simulink model "DJI_Quadcopter_Simulation_2018a"  (R2018a)
settings: Solver=ode45  StartTime=0  StopTime=40  FixedStep=0.02  MaxStep=0.06  RelTol=1e-3  EnableMultiTasking=on
InitFcn:
  | load('batteryModelNew.mat');
  | load('soc_ocv_new.mat');
  | 
  | Q      = battery.QParam; % total capacity in mAh
  | n       = battery.etaParam; % coulombic efficiency
  | M      = battery.MParam; % dynamic hysteresis volts factor
  | Mo     = battery.M0Param; % instant hysteresis volts factor
  | Ro     = battery.R0Param; % internal resistance
  | R       = [battery.RCParam(1)]; % diffusion / warburg impedence, pairs with C
  | C       = [battery.RCParam(2)]; % diffusion / warburg impedence, pairs with R
  | g       = battery.GParam;  % gamma, tunes decay in hysteresis
  | dt      = .01; % delta t
  | eod   = battery.EODParam; % final voltage
  | 
  | if length(R) ~= length(C)
  |     error("R and C must be the same length");
  | end
  | 
  | Arc = zeros(length(R));
  | for i = 1:length(R)
  |     Arc(i,i) = exp(-dt/(R(i)*C(i)));
  | end
  | Brc = zeros(length(R), 1);
  | for i = 1:length(R)
  |     Brc(i,1) = 1 - exp(-dt/(R(i)*C(i)));
  | end
  | k = 1; % timestep
  | Io = .1; % current at time k
  | H(k) = exp(-abs((n(k)*Io(k)*g*dt)/Q));
  | 
  | 
  | %Io = current(1:floor(length(current)/2.5));
  | %Io = current;
  | Io = 0.0;
  | 
  | z = 1.0; % soc
  | Ir = zeros(length(R), 1);
  | h = 0.0;
  | v = ones(length(Io));
  | 
  | 
  | soc = zeros(1, length(Io));
  | v = soc;
model workspace (MAT data in the model file):
  Sig = Simulink.Signal
  Sig.DataType = 'auto'
  Sig.Dimensions = -1
  Sig.DimensionsMode = 'auto'
  Sig.Complexity = 'auto'
  Sig.SampleTime = -1
  Sig.SamplingMode = 'auto'
undefined symbols (not defined in the file): IC, Motor, quadModel, soc_ocv
libraries: simulink x5
(part 1 of 2)
Description:
  | This is a configurable quadcopter simulation.
  | This Simulink model demonstates attitude control.
  | 
  | Additional quadcopter modeling and simulation materials available at:
  | github.com/dch33/Quad-Sim
  | 
  | Copyright (C) 2014 D. Hartman, K. Landis, S. Moreno, J. Kim, M. Mehrer
  | 
  | License:
  |     This program is free software: you can redistribute it and/or modify
  |     it under the terms of the GNU LESSER GENERAL PUBLIC LICENSE as published by
  |     the Free Software Foundation, either version 3 of the License, or
  |     (at your option) any later version.
  | 
  |     This program is distributed in the hope that it will be useful,
  |     but WITHOUT ANY WARRANTY; without even the implied warranty of
  |     MERCHANTABILITY or FITNESS FOR A PARTICULAR PURPOSE.  See the
  |     GNU General Public License for more details.
  | 
  |     You should have received a copy of the GNU LESSER GENERAL PUBLIC LICENSE
  |     along with this program.  If not, see <http://www.gnu.org/licenses/>.
settings Model: ModifiedComment=tdarrah -- Tue Jun 04 05:29:55 2019 -- Version 1.39  Creator=David Hartman  LastModifiedBy=tdarrah
settings Model: ModifiedHistory=|
  | tdarrah -- Tue Jun 04 05:29:55 2019 -- Version 1.39
  | 
  | tdarrah -- Tue Jun 04 05:29:55 2019 -- Version 1.39
  | 
  | tdarrah -- Mon Jun 03 18:31:35 2019 -- Version 1.38
  | closed the battery loop
  | 
  | tdarrah -- Mon Jun 03 18:20:30 2019 -- Version 1.37
  | added battery
  | 
  | 
  | tdarrah -- Mon Jun 03 17:58:08 2019 -- Version 1.36
  | incorporated our motors in model
  | 
  | 
  | Sahai Couso -- Fri May 10 11:35:12 2019 -- Version 1.35
  | 
  | Sahai Couso -- Fri May 10 10:41:34 2019 -- Version 1.34
  | 
  | Sahai Couso -- Fri May 10 10:40:52 2019 -- Version 1.33
  | 
  | Sahai Couso -- Fri May 10 10:30:50 2019 -- Version 1.32
  | 
  | Sahai Couso -- Fri May 10 10:24:25 2019 -- Version 1.31
  | 
  | Sahai Couso -- Wed May 08 22:16:35 2019 -- Version 1.30
  | 
  | Sahai Couso -- Wed May 08 22:15:23 2019 -- Version 1.29
  | 
  | Sahai Couso -- Wed May 08 22:14:58 2019 -- Version 1.28
  | 
  | Sahai Couso -- Wed May 08 22:04:36 2019 -- Version 1.27
  | 
  | Sahai Couso -- Wed May 08 22:04:16 2019 -- Version 1.26
  | 
  | Sahai Couso -- Wed May 08 21:57:14 2019 -- Version 1.25
  | 
  | Sahai Couso -- Wed May 08 21:54:04 2019 -- Version 1.24
  | 
  | Sahai Couso -- Wed May 08 21:53:17 2019 -- Version 1.23
  | 
  | Sahai Couso -- Wed May 08 21:48:07 2019 -- Version 1.22
  | 
  | Sahai Couso -- Wed May 08 21:35:53 2019 -- Version 1.21
  | 
  | Sahai Couso -- Wed May 08 21:28:21 2019 -- Version 1.19
  | 
  | Sahai Couso -- Wed May 08 21:28:21 2019 -- Version 1.19
  | 
  | Sahai Couso -- Wed May 08 21:25:30 2019 -- Version 1.18
  | 
  | Sahai Couso -- Wed May 08 21:23:06 2019 -- Version 1.17
  | 
  | Sahai Couso -- Wed May 08 13:57:34 2019 -- Version 1.16
  | 
  | Sahai Couso -- Wed May 08 00:58:43 2019 -- Version 1.15
  | 
  | Sahai Couso -- Wed May 08 00:58:03 2019 -- Version 1.14
  | 
  | Sahai Couso -- Tue May 07 23:55:58 2019 -- Version 1.13
  | 
  | Sahai Couso -- Tue May 07 23:08:00 2019 -- Version 1.12
  | 
  | Sahai Couso -- Tue May 07 23:06:52 2019 -- Version 1.11
  | 
  | Sahai Couso -- Tue May 07 22:57:09 2019 -- Version 1.10
  | 
  | Sahai Couso -- Tue May 07 22:48:57 2019 -- Version 1.9
  | 
  | Sahai Couso -- Tue May 07 21:40:08 2019 -- Version 1.8
  | 
  | Yves -- Tue Apr 04 13:12:37 2017 -- Version 1.7
  | 
  | Yves -- Tue Apr 04 13:10:33 2017 -- Version 1.6
  | 
  | davidhartman -- Fri Jun 06 23:19:51 2014 -- Version 1.5
  | 
  | 
  | davidhartman -- Fri Jun 06 22:53:10 2014 -- Version 1.3
settings SolverCC: AutoInsertRateTranBlk=on
settings DataIOCC: SaveFormat=Array  SignalLogging=off
settings OptimizationCC: DefaultParameterBehavior=Inlined  LifeSpan=inf
settings DebuggingCC: UnderspecifiedInitializationDetection=Classic  MergeDetectMultiDrivingBlocksExec=none  SolverPrmCheckMsg=warning  UniqueDataStoreMsg=warning  StateNameClashWarn=warning  StrictBusMsg=WarnOnBusTreatedAsVector  SFUnexpectedBacktrackingDiag=warning  SFNoUnconditionalDefaultTransitionDiag=warning  SFExecutionAtInitializationDiag=none
settings HardwareCC: ProdBitPerPointer=32  ProdBitPerSizeT=32  ProdBitPerPtrDiffT=32  ProdLargestAtomicFloat=None  ProdIntDivRoundTo=Undefined  ProdEndianess=Unspecified  ProdWordSize=32  ProdHWDeviceType=32-bit Generic
settings ModelReferenceCC: PropagateSignalLabelsOutOfModel=off
settings CodeAppCC: StateflowObjectComments=on
settings GRTTargetCC: TargetLangStandard=C89/C90 (ANSI)  GeneratePreprocessorConditionals=Disable all
settings ConfigComp: CovMetricSettings=dw  CovHtmlReporting=on  CovSaveCumulativeToWorkspaceVar=on  CovSaveSingleToWorkspaceVar=on  CovExternalEMLEnable=off

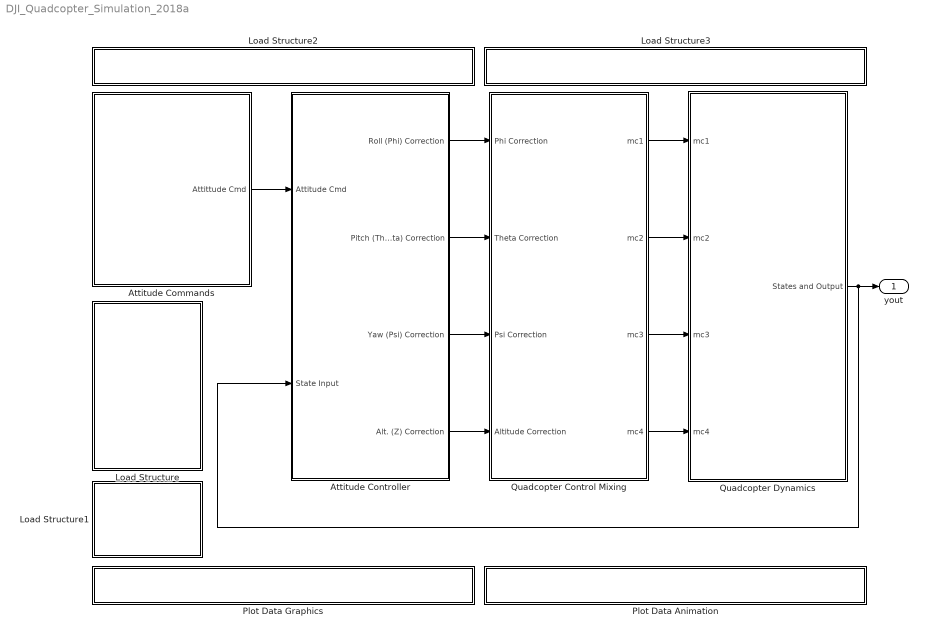
== system DJI_Quadcopter_Simulation_2018a ==
  Attitude Commands : Subsystem
  Attitude Controller : Subsystem
  Load Structure : Subsystem
      settings: OpenFcn=|
      | uiopen('load')
      | if (exist('IC')==1 && exist('quadModel')==1)
      | set_param(bdroot, 'SimulationCommand', 'update')
      | end
      mask Display: fprintf('LOAD:\nQuadcopter\nModel Or\nInitial\nConditions');
  Load Structure1 : Subsystem
      settings: OpenFcn=|
      | if (exist('IC')==1 && exist('quadModel')==1 && exist('yout') && exist('tout'))
      | saveSimResults()
      | else
      | msgbox('No Data To Save!')
      | end
      mask Display: fprintf('SAVE:\nSimulation\nResults');
  Load Structure2 : Subsystem
      settings: OpenFcn=|
      | if exist('GUI_Modeling') == 2,
      | run('GUI_Modeling')
      | 
      | else
      | 
      | msgbox('The desired GUI must be first added to MATLABs path.')
      | 
      | end
      mask Display: fprintf('OPEN GUI: Build New \n Model');
  Load Structure3 : Subsystem
      settings: OpenFcn=|
      | if exist('GUI_IC') == 2,
      | run('GUI_IC')
      | 
      | else
      | 
      | msgbox('The desired GUI must be first added to MATLABs path.')
      | 
      | end
      mask Display: fprintf('OPEN GUI: Create Initial \n Conditions');
  Plot Data Animation : Subsystem
      settings: OpenFcn=|
      | if exist('QuadAnim4') == 2,
      |     if exist('yout')
      | 	run('QuadAnim4');
      |     else
      |     msgbox('Simulation must be run before data can be plotted.');
      |     end
      | else                                                                          msgbox('The desired GUI must be first added to MATLABs path.')
      | end
      mask Display: fprintf('OPEN GUI: Flight Animation')
  Plot Data Graphics : Subsystem
      settings: OpenFcn=|
      | if exist('yout')
      | yout = evalin('base', 'yout');
      | tout = evalin('base', 'tout');
      | quadPlots(yout, tout)
      | else
      | msgbox('Simulation must be run before data can be plotted.')
      | end
      mask Display: fprintf('OPEN PLOT: State Data')
  Quadcopter Control Mixing : Subsystem
      mask Display:
      | modelLoaded = evalin('base','exist(''quadModel'',''var'')');
      | if (modelLoaded==1)
      |     if (evalin('base','quadModel.plusConfig'))
      |     fprintf([' \n' ' \n'  'Configuration "+"']);
      |     else if (~evalin('base','quadModel.plusConfig'))
      |         fprintf([' \n' ' \n' 'Configuration "X"']);
      |         end
      |     end
      | else
      |     fprintf([' \n' ' \n'  'Model Not Loaded']);
      | end
  Quadcopter Dynamics : Subsystem
  yout : Outport
  wires:
  Quadcopter Dynamics/1(States and Output) -> yout/1, Attitude Controller/2(State Input)
  Quadcopter Control Mixing/1(mc1) -> Quadcopter Dynamics/1(mc1)
  Quadcopter Control Mixing/2(mc2) -> Quadcopter Dynamics/2(mc2)
  Quadcopter Control Mixing/3(mc3) -> Quadcopter Dynamics/3(mc3)
  Quadcopter Control Mixing/4(mc4) -> Quadcopter Dynamics/4(mc4)
  Attitude Controller/1(Roll (Phi) Correction) -> Quadcopter Control Mixing/1(Phi Correction)
  Attitude Controller/2(Pitch (Theta) Correction) -> Quadcopter Control Mixing/2(Theta Correction)
  Attitude Controller/3(Yaw (Psi) Correction) -> Quadcopter Control Mixing/3(Psi Correction)
  Attitude Controller/4(Alt. (Z) Correction) -> Quadcopter Control Mixing/4(Altitude Correction)
  Attitude Commands/1(Attittude Cmd) -> Attitude Controller/1(Attitude Cmd)

== system DJI_Quadcopter_Simulation_2018a/Attitude Commands ==
  Bus Creator : BusCreator  Inputs=4
  Step : Step  Time=4  After=-10*pi/180  SampleTime=0
  Step1 : Step  After=10*pi/180  SampleTime=0
  Step2 : Step  Time=7  After=45*pi/180  SampleTime=0
  Step3 : Step  Time=0  Before=10*0.3048  After=10*0.3048  SampleTime=0
  Attittude Cmd : Outport
  tag scope: A=global
  wires:
  Bus Creator/1 -> Attittude Cmd/1, [A]  "Attitude_Cmd"
  Step3/1 -> Bus Creator/4  "Alt_cmd"
  Step2/1 -> Bus Creator/3  "Psi_cmd"
  Step1/1 -> Bus Creator/2  "The_cmd"
  Step/1 -> Bus Creator/1  "Phi_cmd"

== system DJI_Quadcopter_Simulation_2018a/Attitude Controller ==
  Attitude Cmd : Inport
  State Input : Inport  Port=2
  Altitude (Z) Control : Subsystem  mask{Kpz=2, Kiz=1.1, Kdz=3.3, LimitOutput=on, USat=1, LSat=-1, GOffset=(sqrt((quadModel.mass*quadModel.g)/(4*quadModel.ct))-quadModel.b)/quadModel.cr}
      mask prompts: Kpz "Kp"; Kiz "Ki"; Kdz "Kd"; LimitOutput "Integral Saturation?"; USat "Upper saturation limit:"; LSat "Lower saturation limit:"; GOffset "Gravity Feedforward"
      mask help:
      | Adjust PID controller gains through this mask interface, or "look under mask" for more detailed adjustments.
      |
      | Note: Gravity Offset will not appear on block face as a value until simulation is run if it is the result of a formula involving the quadcopter model parameters.
      mask TypeOptions Kpz: Kpz/Gain
      mask TypeOptions Kiz: Kiz/Gain
      mask TypeOptions Kdz: Kdz/Gain
      mask TypeOptions LimitOutput:
      | Integrator
      | Limited/LimitOutput
      mask TypeOptions USat:
      | Integrator
      | Limited/UpperSaturationLimit
      mask TypeOptions LSat:
      | Integrator
      | Limited/LowerSaturationLimit
      mask TypeOptions GOffset: Gravity Offset (Level Flight)/Value
      mask Display:
      | fprintf(['Gravity Offset = ' num2str(GOffset) '\n' ...
      |     'Kp = ' num2str(Kpz) '\n' ...
      |     'Ki = ' num2str(Kiz) '\n' ...
      |     'Kd = ' num2str(Kdz) '\n' ...
      |     'Integral Saturation: ' LimitOutput]);
      | if strcmp(LimitOutput,'on')
      |     fprintf([' \n' ' \n' ' \n' ' \n' ' \n' '\n' ...
      |         'Limits: ' num2str(USat) ' to ' num2str(LSat)]);
      | end
  Bus Selector : BusSelector  OutputSignals=Phi,P,The,Q,Psi,R,Z
  Pitch (Theta) Control : Subsystem  mask{Kpt=2, Kit=1.1, Kdt=1.2, LimitOutput=on, USat=1, LSat=-1}
      mask prompts: Kpt "Kp"; Kit "Ki"; Kdt "Kd"; LimitOutput "Integral Saturation?"; USat "Upper saturation limit:"; LSat "Lower saturation limit:"
      mask help: Adjust PID controller gains through this mask interface, or "look under mask" for more detailed adjustments.
      mask TypeOptions Kpt: Kpt/Gain
      mask TypeOptions Kit: Kit/Gain
      mask TypeOptions Kdt: Kdt/Gain
      mask TypeOptions LimitOutput:
      | Integrator
      | Limited/LimitOutput
      mask TypeOptions USat:
      | Integrator
      | Limited/UpperSaturationLimit
      mask TypeOptions LSat:
      | Integrator
      | Limited/LowerSaturationLimit
      mask Display:
      | fprintf(['Kp = ' num2str(Kpt) '\n' ...
      |     'Ki = ' num2str(Kit) '\n' ...
      |     'Kd = ' num2str(Kdt) '\n' ...
      |     'Integral Saturation: ' LimitOutput]);
      | if strcmp(LimitOutput,'on')
      |     fprintf([' \n' ' \n' ' \n' ' \n' '\n' ...
      |         'Limits: ' num2str(USat) ' to ' num2str(LSat)]);
      | end
  "Roll (Phi) Control " : Subsystem  mask{Kpp=2.0, Kip=1.1, Kdp=1.2, LimitOutput=on, USat=1, LSat=-1}
      mask prompts: Kpp "Kp"; Kip "Ki"; Kdp "Kd"; LimitOutput "Integral Saturation:"; USat "Upper saturation limit:"; LSat "Lower saturation limit:"
      mask help:
      | Adjust PID controller gains through this mask interface, or "look under mask"
      | for more detailed adjustments.
      mask TypeOptions Kpp: Kpp/Gain
      mask TypeOptions Kip: Kip/Gain
      mask TypeOptions Kdp: Kdp/Gain
      mask TypeOptions LimitOutput:
      | Integrator
      | Limited/LimitOutput
      mask TypeOptions USat:
      | Integrator
      | Limited/UpperSaturationLimit
      mask TypeOptions LSat:
      | Integrator
      | Limited/LowerSaturationLimit
      mask Display:
      | fprintf(['Kp = ' num2str(Kpp) '\n' ...
      |     'Ki = ' num2str(Kip) '\n' ...
      |     'Kd = ' num2str(Kdp) '\n'...
      |     'Integral Saturation: ' LimitOutput]);
      | if strcmp(LimitOutput,'on')
      |     fprintf([' \n' ' \n' ' \n' ' \n' '\n' ...
      |         'Limits: ' num2str(USat) ' to ' num2str(LSat)]);
      | end
  Yaw (Psi) Control : Subsystem  mask{Kps=4, Kis=0.5, Kds=3.5, LimitOutput=on, USat=1, LSat=-1}
      mask prompts: Kps "Kp"; Kis "Ki"; Kds "Kd"; LimitOutput "Integral Saturation?"; USat "Upper saturation limit:"; LSat "Lower saturation limit:"
      mask help: Adjust PID controller gains through this mask interface, or "look under mask" for more detailed adjustments.
      mask TypeOptions Kps: Kps/Gain
      mask TypeOptions Kis: Kit/Gain
      mask TypeOptions Kds: Kds/Gain
      mask TypeOptions LimitOutput:
      | Integrator
      | Limited/LimitOutput
      mask TypeOptions USat:
      | Integrator
      | Limited/UpperSaturationLimit
      mask TypeOptions LSat:
      | Integrator
      | Limited/LowerSaturationLimit
      mask Display:
      | fprintf(['Kp = ' num2str(Kps) '\n' ...
      |     'Ki = ' num2str(Kis) '\n' ...
      |     'Kd = ' num2str(Kds) '\n' ...
      |     'Integral Saturation: ' LimitOutput]);
      | if strcmp(LimitOutput,'on')
      |     fprintf([' \n' ' \n' ' \n' ' \n' '\n' ...
      |         'Limits: ' num2str(USat) ' to ' num2str(LSat)]);
      | end
  Roll (Phi) Correction : Outport
  Pitch (Theta) Correction : Outport  Port=2
  Yaw (Psi) Correction : Outport  Port=3
  Alt. (Z) Correction : Outport  Port=4
  wires:
  Bus Selector/6 -> Yaw (Psi) Control/3(R State)  "<R>"
  Bus Selector/4 -> Pitch (Theta) Control/3(Q State)  "<Q>"
  Bus Selector/2 -> "Roll (Phi) Control "/3(P)  "<P>"
  Bus Selector/3 -> Pitch (Theta) Control/2(Theta State)  "<The>"
  Attitude Cmd/1 -> "Roll (Phi) Control "/1("Attitude Command "), Pitch (Theta) Control/1(Attitude Command), Yaw (Psi) Control/1(Attitude Command), Altitude (Z) Control/1(Desired Z)
  Bus Selector/7 -> Altitude (Z) Control/2(Z State)  "<Z>"
  Altitude (Z) Control/1(Alt. (Z) Correction) -> Alt. (Z) Correction/1
  Bus Selector/5 -> Yaw (Psi) Control/2(Psi State)  "<Psi>"
  Yaw (Psi) Control/1(Psi Correction) -> Yaw (Psi) Correction/1
  Pitch (Theta) Control/1(Theta Correction) -> Pitch (Theta) Correction/1
  State Input/1 -> Bus Selector/1
  Bus Selector/1 -> "Roll (Phi) Control "/2(Phi State)  "<Phi>"
  "Roll (Phi) Control "/1(Phi Correction) -> Roll (Phi) Correction/1

== system DJI_Quadcopter_Simulation_2018a/Load Structure ==

== system DJI_Quadcopter_Simulation_2018a/Load Structure1 ==

== system DJI_Quadcopter_Simulation_2018a/Load Structure2 ==

== system DJI_Quadcopter_Simulation_2018a/Load Structure3 ==

== system DJI_Quadcopter_Simulation_2018a/Plot Data Animation ==

== system DJI_Quadcopter_Simulation_2018a/Plot Data Graphics ==

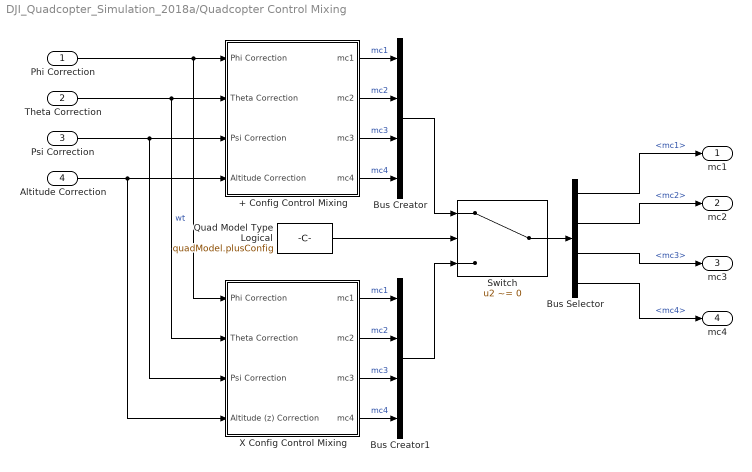
== system DJI_Quadcopter_Simulation_2018a/Quadcopter Control Mixing ==
  Phi Correction : Inport
  Theta Correction : Inport  Port=2
  Psi Correction : Inport  Port=3
  Altitude Correction : Inport  Port=4
  + Config Control Mixing : Subsystem
  Bus Creator : BusCreator  Inputs=4
  Bus Creator1 : BusCreator  Inputs=4
  Bus Selector : BusSelector  OutputSignals=mc1,mc2,mc3,mc4
  Quad Model Type Logical : Constant  Value=quadModel.plusConfig
  Switch : Switch  Criteria=u2 ~= 0
  X Config Control Mixing : Subsystem
  mc1 : Outport
  mc2 : Outport  Port=2
  mc3 : Outport  Port=3
  mc4 : Outport  Port=4
  wires:
  Switch/1 -> Bus Selector/1
  Quad Model Type Logical/1 -> Switch/2
  Bus Selector/4 -> mc4/1  "<mc4>"
  Bus Selector/3 -> mc3/1  "<mc3>"
  Bus Selector/2 -> mc2/1  "<mc2>"
  Bus Selector/1 -> mc1/1  "<mc1>"
  Bus Creator1/1 -> Switch/3
  X Config Control Mixing/4(mc4) -> Bus Creator1/4  "mc4"
  X Config Control Mixing/3(mc3) -> Bus Creator1/3  "mc3"
  X Config Control Mixing/2(mc2) -> Bus Creator1/2  "mc2"
  X Config Control Mixing/1(mc1) -> Bus Creator1/1  "mc1"
  Bus Creator/1 -> Switch/1
  + Config Control Mixing/4(mc4) -> Bus Creator/4  "mc4"
  + Config Control Mixing/3(mc3) -> Bus Creator/3  "mc3"
  + Config Control Mixing/2(mc2) -> Bus Creator/2  "mc2"
  + Config Control Mixing/1(mc1) -> Bus Creator/1  "mc1"
  Altitude Correction/1 -> + Config Control Mixing/4(Altitude Correction), X Config Control Mixing/4(Altitude (z) Correction)
  Psi Correction/1 -> + Config Control Mixing/3(Psi Correction), X Config Control Mixing/3(Psi Correction)
  Theta Correction/1 -> + Config Control Mixing/2(Theta Correction), X Config Control Mixing/2(Theta Correction)  "wt"
  Phi Correction/1 -> + Config Control Mixing/1(Phi Correction), X Config Control Mixing/1(Phi Correction)

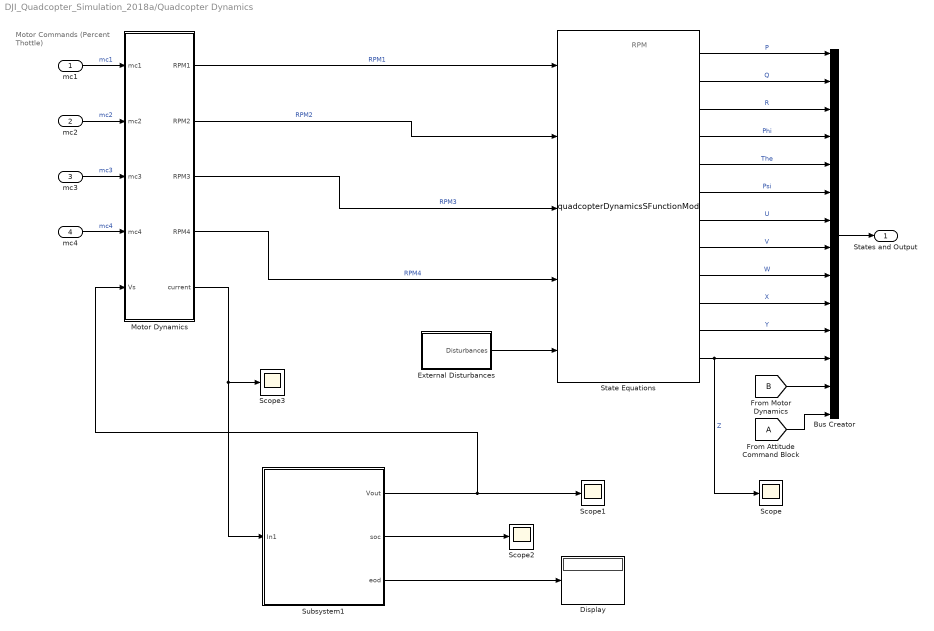
== system DJI_Quadcopter_Simulation_2018a/Quadcopter Dynamics ==
  note: Motor Commands
      | (Percent Thottle)
  note: RPM
  mc1 : Inport
  mc2 : Inport  Port=2
  mc3 : Inport  Port=3
  mc4 : Inport  Port=4
  Bus Creator : BusCreator  Inputs='P','Q','R','Phi','The','Psi','U','V','W','X','Y','Z','mc and RPM','Attitude_Cmd'
  Display : Display
  External Disturbances : Subsystem
  Motor Dynamics : Subsystem
  Scope{,1..3} (4 alike) : Scope
  State Equations : M-S-Function  FunctionName=quadcopterDynamicsSFunctionMod  Parameters=quadModel, IC
      mask Display:
      | port_label('input', 1, 'RPM1')
      | port_label('input', 2, 'RPM2')
      | port_label('input', 3, 'RPM3')
      | port_label('input', 4, 'RPM4')
      | port_label('input', 5, 'Disturbances')
      | port_label('output', 1, 'P')
      | port_label('output', 2, 'Q')
      | port_label('output', 3, 'R')
      | port_label('output', 4, 'Phi')
      | port_label('output', 5, 'The')
      | port_label('output', 6, 'Psi')
      | port_label('output', 7, 'U')
      | port_label('output', 8, 'V')
      | port_label('output', 9, 'W')
      | port_label('output', 10, 'X')
      | port_label('output', 11, 'Y')
      | port_label('output', 12, 'Z')
  Subsystem1 : Subsystem
  States and Output : Outport
  wires:
  [B] -> Bus Creator/13
  [A] -> Bus Creator/14
  External Disturbances/1("Disturbances ") -> State Equations/5
  mc2/1 -> Motor Dynamics/2(mc2)  "mc2"
  mc3/1 -> Motor Dynamics/3(mc3)  "mc3"
  mc4/1 -> Motor Dynamics/4(mc4)  "mc4"
  mc1/1 -> Motor Dynamics/1(mc1)  "mc1"
  Motor Dynamics/4(RPM4) -> State Equations/4  "RPM4"
  Motor Dynamics/3(RPM3) -> State Equations/3  "RPM3"
  Motor Dynamics/2(RPM2) -> State Equations/2  "RPM2"
  Motor Dynamics/1(RPM1) -> State Equations/1  "RPM1"
  Bus Creator/1 -> States and Output/1
  State Equations/12 -> Scope/1, Bus Creator/12  "Z"
  State Equations/11 -> Bus Creator/11  "Y"
  State Equations/10 -> Bus Creator/10  "X"
  State Equations/9 -> Bus Creator/9  "W"
  State Equations/8 -> Bus Creator/8  "V"
  State Equations/7 -> Bus Creator/7  "U"
  State Equations/6 -> Bus Creator/6  "Psi"
  State Equations/5 -> Bus Creator/5  "The"
  State Equations/4 -> Bus Creator/4  "Phi"
  State Equations/3 -> Bus Creator/3  "R"
  State Equations/2 -> Bus Creator/2  "Q"
  State Equations/1 -> Bus Creator/1  "P"
  Subsystem1/1(Vout) -> Motor Dynamics/5(Vs), Scope1/1
  Subsystem1/2(soc) -> Scope2/1
  Subsystem1/3(eod) -> Display/1
  Motor Dynamics/5(current) -> Scope3/1, Subsystem1/1(In1)

== system DJI_Quadcopter_Simulation_2018a/Attitude Controller/Altitude (Z) Control ==
  note: ez
  note: Improve to use rotation matrix and euler angles...
      | maybe with saturation?
  Desired Z : Inport
  Z State : Inport  Port=2
  Bus Selector : BusSelector  OutputSignals=Alt_cmd
  Derivative : Derivative
  Gravity Offset (Level Flight) : Constant  Value=GOffset
  Integrator Limited : Integrator  LimitOutput=on  UpperSaturationLimit=USat  LowerSaturationLimit=LSat
  Kdz : Gain  Gain=Kdz
  Kiz : Gain  Gain=Kiz
  Kpz : Gain  Gain=Kpz
  Scope : Scope
  Scope1 : Scope
  Scope2 : Scope
  Sum : Sum  Inputs=|+-
  Sum2 : Sum  Inputs=+++-
  Alt. (Z) Correction : Outport
  wires:
  Derivative/1 -> Kdz/1
  Bus Selector/1 -> Sum/1  "<Alt_cmd>"
  Integrator Limited/1 -> Kiz/1
  Kdz/1 -> Sum2/4  "D Corr"
  Kiz/1 -> Sum2/3  "I Corr"
  Sum/1 -> Scope/1, Kpz/1, Integrator Limited/1  "Error"
  Kpz/1 -> Sum2/2  "P Corr"
  Sum2/1 -> Scope1/1, Alt. (Z) Correction/1
  Z State/1 -> Sum/2, Derivative/1
  Desired Z/1 -> Bus Selector/1
  Gravity Offset (Level Flight)/1 -> Scope2/1, Sum2/1

== system DJI_Quadcopter_Simulation_2018a/Attitude Controller/Pitch (Theta) Control ==
  Attitude Command : Inport
  Theta State : Inport  Port=2
  Q State : Inport  Port=3
  Bus Selector : BusSelector  OutputSignals=The_cmd
  Integrator Limited : Integrator  LimitOutput=on  UpperSaturationLimit=USat  LowerSaturationLimit=LSat
  Kdt : Gain  Gain=Kdt
  Kit : Gain  Gain=Kit
  Kpt : Gain  Gain=Kpt
  Sum : Sum  Inputs=|+-
  Sum1 : Sum  Inputs=++-
  Theta Correction : Outport
  wires:
  Q State/1 -> Kdt/1
  Bus Selector/1 -> Sum/1  "<The_cmd>"
  Integrator Limited/1 -> Kit/1
  Kit/1 -> Sum1/2  "I Corr"
  Kdt/1 -> Sum1/3  "D Corr"
  Kpt/1 -> Sum1/1  "P Corr"
  Sum1/1 -> Theta Correction/1
  Theta State/1 -> Sum/2
  Attitude Command/1 -> Bus Selector/1
  Sum/1 -> Kpt/1, Integrator Limited/1  "Error"

== system DJI_Quadcopter_Simulation_2018a/Attitude Controller/Roll (Phi) Control  ==
  "Attitude Command " : Inport
  Phi State : Inport  Port=2
  P : Inport  Port=3
  Bus Selector : BusSelector  OutputSignals=Phi_cmd
  Integrator Limited : Integrator  LimitOutput=on  UpperSaturationLimit=USat  LowerSaturationLimit=LSat
  Kdp : Gain  Gain=Kdp
  Kip : Gain  Gain=Kip
  Kpp : Gain  Gain=Kpp
  Sum : Sum  Inputs=|+-
  Sum1 : Sum  Inputs=++-
  Phi Correction : Outport
  wires:
  P/1 -> Kdp/1
  Bus Selector/1 -> Sum/1  "<Phi_cmd>"
  "Attitude Command "/1 -> Bus Selector/1
  Integrator Limited/1 -> Kip/1
  Kip/1 -> Sum1/2  "I Corr"
  Kdp/1 -> Sum1/3  "D Corr"
  Kpp/1 -> Sum1/1  "P Corr"
  Sum1/1 -> Phi Correction/1
  Phi State/1 -> Sum/2
  Sum/1 -> Kpp/1, Integrator Limited/1  "Error"

== system DJI_Quadcopter_Simulation_2018a/Attitude Controller/Yaw (Psi) Control ==
  Attitude Command : Inport
  Psi State : Inport  Port=2
  R State : Inport  Port=3
  Bus Selector : BusSelector  OutputSignals=Psi_cmd
  Integrator Limited : Integrator  LimitOutput=on  UpperSaturationLimit=USat  LowerSaturationLimit=LSat
  Kds : Gain  Gain=Kds
  Kit : Gain  Gain=Kis
  Kps : Gain  Gain=Kps
  Sum : Sum  Inputs=|+-
  Sum1 : Sum  Inputs=++-
  Psi Correction : Outport
  wires:
  R State/1 -> Kds/1
  Bus Selector/1 -> Sum/1  "<Psi_cmd>"
  Integrator Limited/1 -> Kit/1
  Kit/1 -> Sum1/2  "I Corr"
  Kds/1 -> Sum1/3  "D Corr"
  Kps/1 -> Sum1/1  "P Corr"
  Psi State/1 -> Sum/2
  Sum1/1 -> Psi Correction/1
  Attitude Command/1 -> Bus Selector/1
  Sum/1 -> Kps/1, Integrator Limited/1  "Error"

== system DJI_Quadcopter_Simulation_2018a/Quadcopter Control Mixing/+ Config Control Mixing ==
  note: mc1 = Alt_cor -Psi_cor - The_cor
  note: mc3 = Alt_cor - Psi_cor + The_cor
  note: mc4 = Alt_cor + Psi_cor - Phi_cor
  note: + (plus) Quad Configuration Control Mixing
  note: mc2 = Alt_cor + Psi_cor + Phi_cor
  Phi Correction : Inport
  Theta Correction : Inport  Port=2
  Psi Correction : Inport  Port=3
  Altitude Correction : Inport  Port=4
  Sum1 : Sum  Inputs=|+-
  Sum11 : Sum  Inputs=-+|
  Sum2 : Sum  Inputs=|+-
  Sum3 : Sum  Inputs=++|
  Sum4 : Sum  Inputs=++|
  Sum8 : Sum  Inputs=|++
  mc1 : Outport
  mc2 : Outport  Port=2
  mc3 : Outport  Port=3
  mc4 : Outport  Port=4
  wires:
  Sum11/1 -> mc4/1
  Sum8/1 -> mc2/1
  Sum3/1 -> mc3/1
  Sum1/1 -> mc1/1
  Phi Correction/1 -> Sum11/1, Sum8/2
  Sum4/1 -> Sum8/1, Sum11/2
  Psi Correction/1 -> Sum2/2, Sum4/1
  Sum2/1 -> Sum1/1, Sum3/2
  Altitude Correction/1 -> Sum4/2, Sum2/1
  Theta Correction/1 -> Sum3/1, Sum1/2

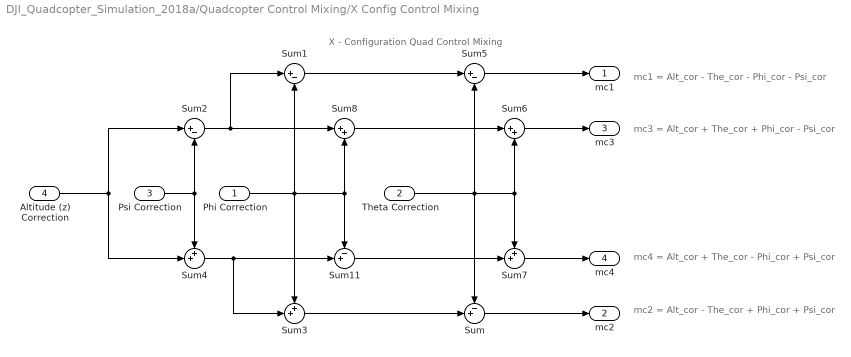
== system DJI_Quadcopter_Simulation_2018a/Quadcopter Control Mixing/X Config Control Mixing ==
  note: mc4 = Alt_cor + The_cor - Phi_cor + Psi_cor
  note: mc2 = Alt_cor - The_cor + Phi_cor + Psi_cor
  note: mc3 = Alt_cor + The_cor + Phi_cor - Psi_cor
  note: X - Configuration Quad Control Mixing
  note: mc1 = Alt_cor - The_cor - Phi_cor - Psi_cor
  Phi Correction : Inport
  Theta Correction : Inport  Port=2
  Psi Correction : Inport  Port=3
  Altitude (z) Correction : Inport  Port=4
  Sum : Sum  Inputs=-+|
  Sum1 : Sum  Inputs=|+-
  Sum11 : Sum  Inputs=-+|
  Sum2 : Sum  Inputs=|+-
  Sum3 : Sum  Inputs=++|
  Sum4 : Sum  Inputs=++|
  Sum5 : Sum  Inputs=|+-
  Sum6 : Sum  Inputs=|++
  Sum7 : Sum  Inputs=++|
  Sum8 : Sum  Inputs=|++
  mc1 : Outport
  mc2 : Outport  Port=2
  mc3 : Outport  Port=3
  mc4 : Outport  Port=4
  wires:
  Sum/1 -> mc2/1
  Altitude (z) Correction/1 -> Sum4/2, Sum2/1
  Sum7/1 -> mc4/1
  Sum6/1 -> mc3/1
  Sum5/1 -> mc1/1
  Sum11/1 -> Sum7/2
  Sum8/1 -> Sum6/1
  Sum1/1 -> Sum5/1
  Theta Correction/1 -> Sum/1, Sum5/2, Sum6/2, Sum7/1
  Sum3/1 -> Sum/2
  Sum4/1 -> Sum11/2, Sum3/2
  Phi Correction/1 -> Sum11/1, Sum8/2, Sum1/2, Sum3/1
  Psi Correction/1 -> Sum2/2, Sum4/1
  Sum2/1 -> Sum1/1, Sum8/1

== system DJI_Quadcopter_Simulation_2018a/Quadcopter Dynamics/External Disturbances ==
  note: Note: Torques are in units of N*m, Forces in N
      | Torques are applied to the BODY coordinate system.
      | Forces are applied from the WORLD coordinate system!
      | This can be changed by adjusting the equations within the S-function.
  Bus Creator : BusCreator  Inputs=6
  Bus to Vector : BusToVector
  Constant{2..6} (5 alike) : Constant  Value=0
  Step : Step  After=0  SampleTime=0
  "Disturbances " : Outport
  wires:
  Constant5/1 -> Bus Creator/6  "Force_z-axis"
  Constant4/1 -> Bus Creator/5  "Force_y-axis"
  Constant3/1 -> Bus Creator/4  "Force_x-axis"
  Constant2/1 -> Bus Creator/3  "Tau_bz-axis"
  Step/1 -> Bus Creator/2  "Tau_by-axis"
  Constant6/1 -> Bus Creator/1  "Tau_bx-axis"
  Bus Creator/1 -> Bus to Vector/1
  Bus to Vector/1 -> "Disturbances "/1

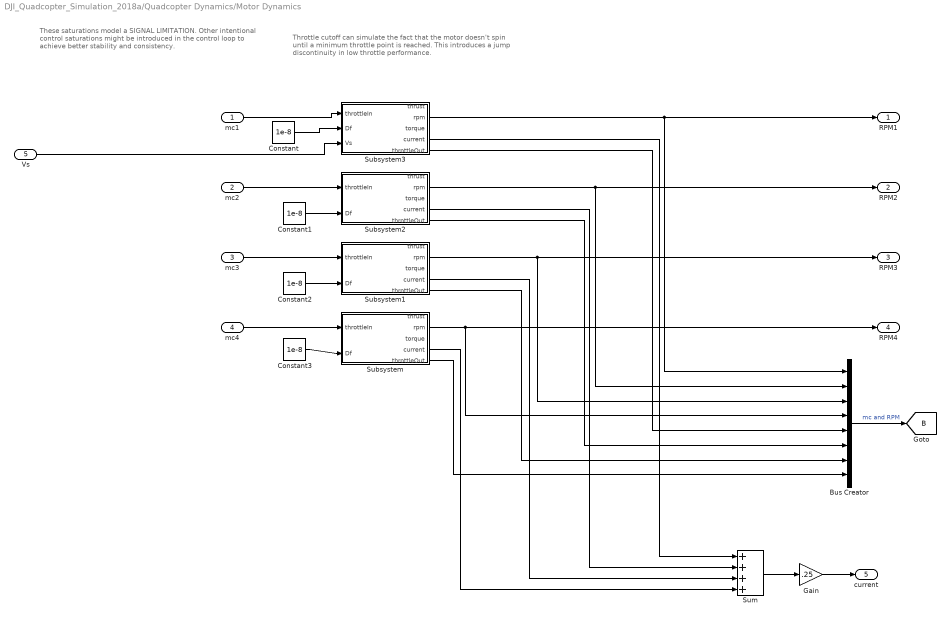
== system DJI_Quadcopter_Simulation_2018a/Quadcopter Dynamics/Motor Dynamics ==
  note: These saturations model a SIGNAL LIMITATION.
      | Other intentional control saturations might be introduced in the
      | control loop to achieve better stability and consistency.
  note: Throttle cutoff can simulate the fact that the motor doesn't
      | spin until a minimum throttle point is reached. This introduces
      | a jump discontinuity in low throttle performance.
  mc1 : Inport
  mc2 : Inport  Port=2
  mc3 : Inport  Port=3
  mc4 : Inport  Port=4
  Vs : Inport  Port=5
  Bus Creator : BusCreator  Inputs=8
  Constant{,1..3} (4 alike) : Constant  Value=1e-8
  Gain : Gain  Gain=.25
  Subsystem : Subsystem
  Subsystem1 : Subsystem
  Subsystem2 : Subsystem
  Subsystem3 : Subsystem
  Sum : Sum  Inputs=++++
  RPM1 : Outport
  RPM2 : Outport  Port=2
  RPM3 : Outport  Port=3
  RPM4 : Outport  Port=4
  current : Outport  Port=5
  tag scope: B=global
  wires:
  Bus Creator/1 -> [B]  "mc and RPM"
  Subsystem3/2(rpm) -> RPM1/1, Bus Creator/1
  mc1/1 -> Subsystem3/1(throttleIn)
  Constant/1 -> Subsystem3/2(Df)
  Subsystem3/5(throttleOut) -> Bus Creator/5
  Subsystem2/2(rpm) -> RPM2/1, Bus Creator/2
  mc2/1 -> Subsystem2/1(throttleIn)
  Constant1/1 -> Subsystem2/2(Df)
  Subsystem2/5(throttleOut) -> Bus Creator/6
  Subsystem1/2(rpm) -> Bus Creator/3, RPM3/1
  mc3/1 -> Subsystem1/1(throttleIn)
  Constant2/1 -> Subsystem1/2(Df)
  Subsystem1/5(throttleOut) -> Bus Creator/7
  Subsystem/2(rpm) -> RPM4/1, Bus Creator/4
  mc4/1 -> Subsystem/1(throttleIn)
  Constant3/1 -> Subsystem/2(Df)
  Subsystem/5(throttleOut) -> Bus Creator/8
  Subsystem/4(current) -> Sum/4
  Subsystem1/4(current) -> Sum/3
  Subsystem2/4(current) -> Sum/2
  Subsystem3/4(current) -> Sum/1
  Sum/1 -> Gain/1
  Vs/1 -> Subsystem3/3(Vs)
  Gain/1 -> current/1

== system DJI_Quadcopter_Simulation_2018a/Quadcopter Dynamics/Subsystem1 ==
  In1 : Inport
  Constant1 : Constant  Value=0
  Display1 : Display
  Equal : RelationalOperator  Operator===  OutDataTypeStr=boolean  RndMeth=Simplest
  Scope3 : Scope
  Stop Simulation : Stop
  Subsystem : Subsystem
  Vout : Outport
  soc : Outport  Port=2
  eod : Outport  Port=3
  wires:
  Subsystem/1(Vout) -> Vout/1
  Subsystem/2(soc) -> soc/1
  In1/1 -> Equal/1, Scope3/1, Subsystem/1(current)
  Subsystem/3(eod) -> eod/1
  Constant1/1 -> Equal/2
  Equal/1 -> Display1/1, Stop Simulation/1

== system DJI_Quadcopter_Simulation_2018a/Quadcopter Dynamics/Motor Dynamics/Subsystem ==
  throttleIn : Inport
  Df : Inport  Port=2
  Signal_Saturation_4 : Saturate  UpperLimit=100  LowerLimit=0
  Throttle To RPM Gain and Cutoff_8 : Subsystem
  motorRotor4 : Subsystem
  thrust : Outport
  rpm : Outport  Port=2
  torque : Outport  Port=3
  current : Outport  Port=4
  throttleOut : Outport  Port=5
  wires:
  Throttle To RPM Gain and Cutoff_8/1(Out5) -> motorRotor4/1(V)
  motorRotor4/4(current) -> current/1
  motorRotor4/2(rpm) -> rpm/1
  throttleIn/1 -> Signal_Saturation_4/1
  motorRotor4/3(torque) -> torque/1
  motorRotor4/1(thrust) -> thrust/1
  Signal_Saturation_4/1 -> Throttle To RPM Gain and Cutoff_8/1(In5), throttleOut/1
  Df/1 -> motorRotor4/2(Df)

== system DJI_Quadcopter_Simulation_2018a/Quadcopter Dynamics/Motor Dynamics/Subsystem1 ==
  throttleIn : Inport
  Df : Inport  Port=2
  Signal_Saturation_4 : Saturate  UpperLimit=100  LowerLimit=0
  Throttle To RPM Gain and Cutoff_8 : Subsystem
  motorRotor4 : Subsystem
  thrust : Outport
  rpm : Outport  Port=2
  torque : Outport  Port=3
  current : Outport  Port=4
  throttleOut : Outport  Port=5
  wires:
  Throttle To RPM Gain and Cutoff_8/1(Out5) -> motorRotor4/1(V)
  motorRotor4/4(current) -> current/1
  motorRotor4/2(rpm) -> rpm/1
  throttleIn/1 -> Signal_Saturation_4/1
  motorRotor4/3(torque) -> torque/1
  motorRotor4/1(thrust) -> thrust/1
  Signal_Saturation_4/1 -> Throttle To RPM Gain and Cutoff_8/1(In5), throttleOut/1
  Df/1 -> motorRotor4/2(Df)

== system DJI_Quadcopter_Simulation_2018a/Quadcopter Dynamics/Motor Dynamics/Subsystem2 ==
  throttleIn : Inport
  Df : Inport  Port=2
  Signal_Saturation_4 : Saturate  UpperLimit=100  LowerLimit=0
  Throttle To RPM Gain and Cutoff_8 : Subsystem
  motorRotor4 : Subsystem
  thrust : Outport
  rpm : Outport  Port=2
  torque : Outport  Port=3
  current : Outport  Port=4
  throttleOut : Outport  Port=5
  wires:
  Throttle To RPM Gain and Cutoff_8/1(Out5) -> motorRotor4/1(V)
  motorRotor4/4(current) -> current/1
  motorRotor4/2(rpm) -> rpm/1
  throttleIn/1 -> Signal_Saturation_4/1
  motorRotor4/3(torque) -> torque/1
  motorRotor4/1(thrust) -> thrust/1
  Signal_Saturation_4/1 -> Throttle To RPM Gain and Cutoff_8/1(In5), throttleOut/1
  Df/1 -> motorRotor4/2(Df)

== system DJI_Quadcopter_Simulation_2018a/Quadcopter Dynamics/Motor Dynamics/Subsystem3 ==
  note: Throttle cutoff can simulate the fact that the motor doesn't
      | spin until a minimum throttle point is reached. This introduces
      | a jump discontinuity in low throttle performance.
  note: These saturations model a SIGNAL LIMITATION.
      | Other intentional control saturations might be introduced in the
      | control loop to achieve better stability and consistency.
  throttleIn : Inport
  Df : Inport  Port=2
  Vs : Inport  Port=3
  Scope : Scope
  Signal_Saturation_4 : Saturate  UpperLimit=100  LowerLimit=0
  Throttle To RPM Gain and Cutoff_8 : Subsystem
  motorRotor4 : Subsystem
  thrust : Outport
  rpm : Outport  Port=2
  torque : Outport  Port=3
  current : Outport  Port=4
  throttleOut : Outport  Port=5
  wires:
  Throttle To RPM Gain and Cutoff_8/1(Out5) -> motorRotor4/1(V), Scope/1
  motorRotor4/4(current) -> current/1
  motorRotor4/2(rpm) -> rpm/1
  throttleIn/1 -> Signal_Saturation_4/1
  motorRotor4/3(torque) -> torque/1
  motorRotor4/1(thrust) -> thrust/1
  Signal_Saturation_4/1 -> Throttle To RPM Gain and Cutoff_8/1(In5), throttleOut/1
  Df/1 -> motorRotor4/2(Df)
  Vs/1 -> Throttle To RPM Gain and Cutoff_8/2(Vs)

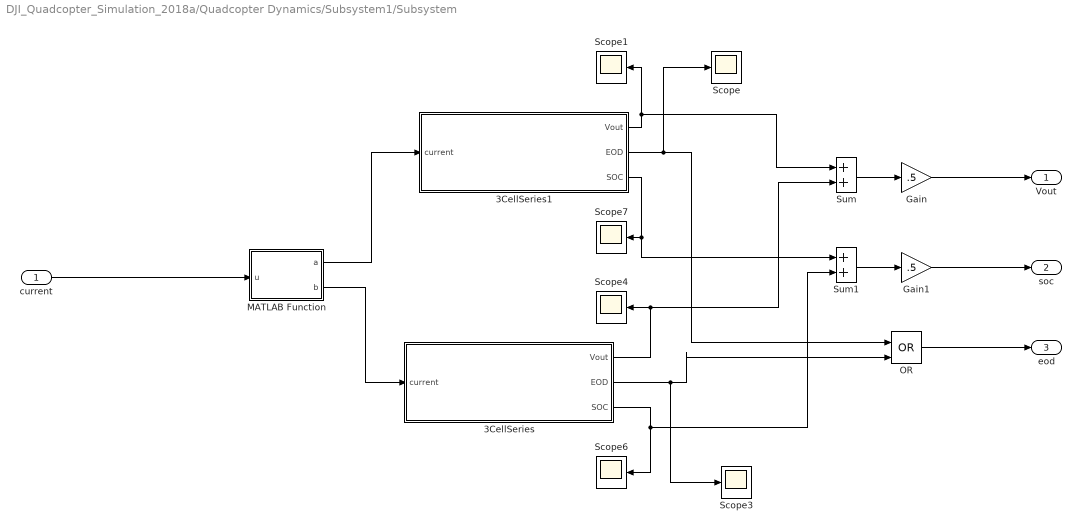
== system DJI_Quadcopter_Simulation_2018a/Quadcopter Dynamics/Subsystem1/Subsystem ==
  current : Inport
  3CellSeries : Subsystem
  3CellSeries1 : Subsystem
  Gain : Gain  Gain=.5
  Gain1 : Gain  Gain=.5
  MATLAB Function : MATLAB Function  TreatAsAtomicUnit=on
  OR : Logic  Operator=OR  IconShape=distinctive  AllPortsSameDT=off  OutDataTypeStr=boolean
  Scope{,1,3..4,6..7} (6 alike) : Scope
  Sum : Sum
  Sum1 : Sum
  Vout : Outport
  soc : Outport  Port=2
  eod : Outport  Port=3
  wires:
  MATLAB Function/2(b) -> 3CellSeries/1(current)
  MATLAB Function/1(a) -> 3CellSeries1/1(current)
  3CellSeries/1(Vout) -> Sum/2, Scope4/1
  Gain/1 -> Vout/1
  3CellSeries1/2(EOD) -> Scope/1, OR/1
  current/1 -> MATLAB Function/1(u)
  3CellSeries1/3(SOC) -> Sum1/1, Scope7/1
  Sum/1 -> Gain/1
  3CellSeries/3(SOC) -> Sum1/2, Scope6/1
  3CellSeries1/1(Vout) -> Sum/1, Scope1/1
  3CellSeries/2(EOD) -> Scope3/1, OR/2
  Sum1/1 -> Gain1/1
  Gain1/1 -> soc/1
  OR/1 -> eod/1

== system DJI_Quadcopter_Simulation_2018a/Quadcopter Dynamics/Motor Dynamics/Subsystem/Throttle To RPM Gain and Cutoff_8 ==
  note: Output equals linearly scaled RPM
      | for given throttle input if throttle input >=Throttle Cuttoff (minThr)
      | else output is zero.
  In5 : Inport
  Constant : Constant  Value=quadModel.VoltMin
  Gain : Gain  Gain=quadModel.VoltSlope
  Minimum Throttle Cutoff : simulink/Logic and Bit Operations/Compare To Constant  relop=>=  const=quadModel.minThr  OutDataTypeStr=uint8
  Product : Product
  Sum1 : Sum  Inputs=++|
  Out5 : Outport
  wires:
  Minimum Throttle Cutoff/1 -> Product/2
  Product/1 -> Out5/1
  In5/1 -> Gain/1, Minimum Throttle Cutoff/1
  Gain/1 -> Sum1/2
  Sum1/1 -> Product/1
  Constant/1 -> Sum1/1

== system DJI_Quadcopter_Simulation_2018a/Quadcopter Dynamics/Motor Dynamics/Subsystem/motorRotor4 ==
  V : Inport
  Df : Inport  Port=2
  Convert rad/s to rmp : Gain  Gain=60/(2*pi)
  Electrical part : Subsystem
  Mechanical part : Subsystem
  thrust : Outport
  rpm : Outport  Port=2
  torque : Outport  Port=3
  current : Outport  Port=4
  wires:
  Convert rad/s to rmp/1 -> rpm/1
  V/1 -> Electrical part/1(ESC voltage)
  Mechanical part/2(Thrust) -> thrust/1
  Electrical part/1(Electrical Torque) -> Mechanical part/2(Electrical Torque)
  Mechanical part/3(Torque) -> torque/1
  Mechanical part/1(w angular speed) -> Electrical part/2(w angular speed), Convert rad/s to rmp/1
  Df/1 -> Mechanical part/1(dynamicFriction)
  Electrical part/2(current) -> current/1

== system DJI_Quadcopter_Simulation_2018a/Quadcopter Dynamics/Motor Dynamics/Subsystem1/Throttle To RPM Gain and Cutoff_8 ==
  note: Output equals linearly scaled RPM
      | for given throttle input if throttle input >=Throttle Cuttoff (minThr)
      | else output is zero.
  In5 : Inport
  Constant : Constant  Value=quadModel.VoltMin
  Gain : Gain  Gain=quadModel.VoltSlope
  Minimum Throttle Cutoff : simulink/Logic and Bit Operations/Compare To Constant  relop=>=  const=quadModel.minThr  OutDataTypeStr=uint8
  Product : Product
  Sum1 : Sum  Inputs=++|
  Out5 : Outport
  wires:
  Minimum Throttle Cutoff/1 -> Product/2
  Product/1 -> Out5/1
  In5/1 -> Gain/1, Minimum Throttle Cutoff/1
  Gain/1 -> Sum1/2
  Sum1/1 -> Product/1
  Constant/1 -> Sum1/1

== system DJI_Quadcopter_Simulation_2018a/Quadcopter Dynamics/Motor Dynamics/Subsystem1/motorRotor4 ==
  V : Inport
  Df : Inport  Port=2
  Convert rad/s to rmp : Gain  Gain=60/(2*pi)
  Electrical part : Subsystem
  Mechanical part : Subsystem
  thrust : Outport
  rpm : Outport  Port=2
  torque : Outport  Port=3
  current : Outport  Port=4
  wires:
  Convert rad/s to rmp/1 -> rpm/1
  V/1 -> Electrical part/1(ESC voltage)
  Mechanical part/2(Thrust) -> thrust/1
  Electrical part/1(Electrical Torque) -> Mechanical part/2(Electrical Torque)
  Mechanical part/3(Torque) -> torque/1
  Mechanical part/1(w angular speed) -> Electrical part/2(w angular speed), Convert rad/s to rmp/1
  Df/1 -> Mechanical part/1(dynamicFriction)
  Electrical part/2(current) -> current/1

== system DJI_Quadcopter_Simulation_2018a/Quadcopter Dynamics/Motor Dynamics/Subsystem2/Throttle To RPM Gain and Cutoff_8 ==
  note: Output equals linearly scaled RPM
      | for given throttle input if throttle input >=Throttle Cuttoff (minThr)
      | else output is zero.
  In5 : Inport
  Constant : Constant  Value=quadModel.VoltMin
  Gain : Gain  Gain=quadModel.VoltSlope
  Minimum Throttle Cutoff : simulink/Logic and Bit Operations/Compare To Constant  relop=>=  const=quadModel.minThr  OutDataTypeStr=uint8
  Product : Product
  Sum1 : Sum  Inputs=++|
  Out5 : Outport
  wires:
  Minimum Throttle Cutoff/1 -> Product/2
  Product/1 -> Out5/1
  In5/1 -> Gain/1, Minimum Throttle Cutoff/1
  Gain/1 -> Sum1/2
  Sum1/1 -> Product/1
  Constant/1 -> Sum1/1

== system DJI_Quadcopter_Simulation_2018a/Quadcopter Dynamics/Motor Dynamics/Subsystem2/motorRotor4 ==
  V : Inport
  Df : Inport  Port=2
  Convert rad/s to rmp : Gain  Gain=60/(2*pi)
  Electrical part : Subsystem
  Mechanical part : Subsystem
  thrust : Outport
  rpm : Outport  Port=2
  torque : Outport  Port=3
  current : Outport  Port=4
  wires:
  Convert rad/s to rmp/1 -> rpm/1
  V/1 -> Electrical part/1(ESC voltage)
  Mechanical part/2(Thrust) -> thrust/1
  Electrical part/1(Electrical Torque) -> Mechanical part/2(Electrical Torque)
  Mechanical part/3(Torque) -> torque/1
  Mechanical part/1(w angular speed) -> Electrical part/2(w angular speed), Convert rad/s to rmp/1
  Df/1 -> Mechanical part/1(dynamicFriction)
  Electrical part/2(current) -> current/1

== system DJI_Quadcopter_Simulation_2018a/Quadcopter Dynamics/Motor Dynamics/Subsystem3/Throttle To RPM Gain and Cutoff_8 ==
  note: Output equals linearly scaled RPM
      | for given throttle input if throttle input >=Throttle Cuttoff (minThr)
      | else output is zero.
  note: Output equals linearly scaled RPM
      | for given throttle input if throttle input >=Throttle Cuttoff (minThr)
      | else output is zero.
  In5 : Inport
  Vs : Inport  Port=2
  Constant1 : Constant  Commented=on  Value=quadModel.VoltMin
  Gain : Gain  Gain=.01
  Gain1 : Gain  Commented=on  Gain=quadModel.VoltSlope
  Minimum Throttle Cutoff : simulink/Logic and Bit Operations/Compare To Constant  relop=>=  const=quadModel.minThr  OutDataTypeStr=uint8
  Minimum Throttle Cutoff1 : simulink/Logic and Bit Operations/Compare To Constant  Commented=on  relop=>=  const=quadModel.minThr  OutDataTypeStr=uint8
  Product : Product
  Product1 : Product  Commented=on
  Product2 : Product
  Sum2 : Sum  Commented=on  Inputs=++|
  Out5 : Outport
  wires:
  Minimum Throttle Cutoff/1 -> Product/2
  Product/1 -> Out5/1
  In5/1 -> Gain/1, Minimum Throttle Cutoff/1
  Gain/1 -> Product2/2
  Product2/1 -> Product/1
  Gain1/1 -> Sum2/2
  Constant1/1 -> Sum2/1
  Sum2/1 -> Product1/1
  Minimum Throttle Cutoff1/1 -> Product1/2
  Vs/1 -> Product2/1

== system DJI_Quadcopter_Simulation_2018a/Quadcopter Dynamics/Motor Dynamics/Subsystem3/motorRotor4 ==
  V : Inport
  Df : Inport  Port=2
  Convert rad/s to rmp : Gain  Gain=60/(2*pi)
  Electrical part : Subsystem
  Mechanical part : Subsystem
  thrust : Outport
  rpm : Outport  Port=2
  torque : Outport  Port=3
  current : Outport  Port=4
  wires:
  Convert rad/s to rmp/1 -> rpm/1
  V/1 -> Electrical part/1(ESC voltage)
  Mechanical part/2(Thrust) -> thrust/1
  Electrical part/1(Electrical Torque) -> Mechanical part/2(Electrical Torque)
  Mechanical part/3(Torque) -> torque/1
  Mechanical part/1(w angular speed) -> Electrical part/2(w angular speed), Convert rad/s to rmp/1
  Df/1 -> Mechanical part/1(dynamicFriction)
  Electrical part/2(current) -> current/1

== system DJI_Quadcopter_Simulation_2018a/Quadcopter Dynamics/Subsystem1/Subsystem/3CellSeries ==
  current : Inport
  Cell4 : Subsystem
  Cell5 : Subsystem
  Cell6 : Subsystem
  Gain : Gain  Gain=1/3
  Mux1 : Mux  Inputs=3
  Stop Simulation : Stop
  Sum2 : Sum  Inputs=+++
  Sum3 : Sum  Inputs=+++
  Vout : Outport
  EOD : Outport  Port=2
  SOC : Outport  Port=3
  wires:
  Sum2/1 -> Vout/1
  Cell5/1(Vout) -> Sum2/2
  Cell6/1(Vout) -> Sum2/3
  current/1 -> Cell6/1(current), Cell5/1(current), Cell4/1(current)
  Mux1/1 -> Stop Simulation/1, EOD/1
  Cell4/2(soc) -> Sum3/1
  Cell6/2(soc) -> Sum3/3
  Cell4/1(Vout) -> Sum2/1
  Cell5/2(soc) -> Sum3/2
  Sum3/1 -> Gain/1
  Gain/1 -> SOC/1
  Cell5/3(EOD) -> Mux1/2  "cell2"
  Cell6/3(EOD) -> Mux1/3  "cell3"
  Cell4/3(EOD) -> Mux1/1  "cell1"

== system DJI_Quadcopter_Simulation_2018a/Quadcopter Dynamics/Subsystem1/Subsystem/3CellSeries1 ==
  current : Inport
  Cell4 : Subsystem
  Cell5 : Subsystem
  Cell6 : Subsystem
  Gain : Gain  Gain=1/3
  Mux1 : Mux  Inputs=3
  Stop Simulation : Stop
  Sum2 : Sum  Inputs=+++
  Sum3 : Sum  Inputs=+++
  Vout : Outport
  EOD : Outport  Port=2
  SOC : Outport  Port=3
  wires:
  Cell6/3(EOD) -> Mux1/3  "cell3"
  Sum2/1 -> Vout/1
  Cell5/1(Vout) -> Sum2/2
  Cell5/3(EOD) -> Mux1/2  "cell2"
  Cell6/1(Vout) -> Sum2/3
  current/1 -> Cell6/1(current), Cell5/1(current), Cell4/1(current)
  Mux1/1 -> Stop Simulation/1, EOD/1
  Cell4/2(soc) -> Sum3/1
  Cell6/2(soc) -> Sum3/3
  Cell4/1(Vout) -> Sum2/1
  Cell5/2(soc) -> Sum3/2
  Sum3/1 -> Gain/1
  Cell4/3(EOD) -> Mux1/1  "cell1"
  Gain/1 -> SOC/1

== system DJI_Quadcopter_Simulation_2018a/Quadcopter Dynamics/Motor Dynamics/Subsystem/motorRotor4/Electrical part ==
  ESC voltage : Inport
  w angular speed : Inport  Port=2
  1/R : Gain  Gain=1/Motor.Req
  Ke (Torque constant)1 : Gain  Gain=Motor.Ke_eq
  Kt (Torque constant) Kt=Ke for an ideal square wave motor : Gain  Gain=Motor.Ke_eq
  Sum : Sum  Inputs=|+-
  Electrical Torque : Outport
  current : Outport  Port=2
  wires:
  1/R/1 -> current/1, Kt (Torque constant) Kt=Ke for an ideal square wave motor/1  "current i"
  Sum/1 -> 1/R/1
  Kt (Torque constant) Kt=Ke for an ideal square wave motor/1 -> Electrical Torque/1
  Ke (Torque constant)1/1 -> Sum/2
  ESC voltage/1 -> Sum/1
  w angular speed/1 -> Ke (Torque constant)1/1

== system DJI_Quadcopter_Simulation_2018a/Quadcopter Dynamics/Motor Dynamics/Subsystem/motorRotor4/Mechanical part ==
  dynamicFriction : Inport
  Electrical Torque : Inport  Port=2
  1/J Inertia constant : Gain  Gain=1/Motor.J
  Convert rad/s to rmp : Gain  Gain=60/(2*pi)
  Integrator : Integrator  InitialCondition=IC.w4
  Product : Product
  "Propeller model " : MATLAB Function  TreatAsAtomicUnit=on
  Sum1 : Sum  Inputs=--+-
  staticFriction : Constant  Value=10e-7
  w angular speed : Outport
  Thrust : Outport  Port=2
  Torque : Outport  Port=3
  wires:
  "Propeller model "/1(torque) -> Sum1/1, Torque/1
  1/J Inertia constant/1 -> Integrator/1
  dynamicFriction/1 -> Product/2
  Product/1 -> Sum1/4
  Integrator/1 -> Product/1, w angular speed/1, Convert rad/s to rmp/1  "w angular speed"
  Sum1/1 -> 1/J Inertia constant/1
  Electrical Torque/1 -> Sum1/3
  Convert rad/s to rmp/1 -> "Propeller model "/1(rpm)
  "Propeller model "/2(thrust) -> Thrust/1
  staticFriction/1 -> Sum1/2

== system DJI_Quadcopter_Simulation_2018a/Quadcopter Dynamics/Motor Dynamics/Subsystem1/motorRotor4/Electrical part ==
  ESC voltage : Inport
  w angular speed : Inport  Port=2
  1/R : Gain  Gain=1/Motor.Req
  Ke (Torque constant)1 : Gain  Gain=Motor.Ke_eq
  Kt (Torque constant) Kt=Ke for an ideal square wave motor : Gain  Gain=Motor.Ke_eq
  Sum : Sum  Inputs=|+-
  Electrical Torque : Outport
  current : Outport  Port=2
  wires:
  1/R/1 -> current/1, Kt (Torque constant) Kt=Ke for an ideal square wave motor/1  "current i"
  Sum/1 -> 1/R/1
  Kt (Torque constant) Kt=Ke for an ideal square wave motor/1 -> Electrical Torque/1
  Ke (Torque constant)1/1 -> Sum/2
  ESC voltage/1 -> Sum/1
  w angular speed/1 -> Ke (Torque constant)1/1

== system DJI_Quadcopter_Simulation_2018a/Quadcopter Dynamics/Motor Dynamics/Subsystem1/motorRotor4/Mechanical part ==
  dynamicFriction : Inport
  Electrical Torque : Inport  Port=2
  1/J Inertia constant : Gain  Gain=1/Motor.J
  Convert rad/s to rmp : Gain  Gain=60/(2*pi)
  Integrator : Integrator  InitialCondition=IC.w4
  Product : Product
  "Propeller model " : MATLAB Function  TreatAsAtomicUnit=on
  Sum1 : Sum  Inputs=--+-
  staticFriction : Constant  Value=10e-7
  w angular speed : Outport
  Thrust : Outport  Port=2
  Torque : Outport  Port=3
  wires:
  "Propeller model "/1(torque) -> Sum1/1, Torque/1
  1/J Inertia constant/1 -> Integrator/1
  dynamicFriction/1 -> Product/2
  Product/1 -> Sum1/4
  Integrator/1 -> Product/1, w angular speed/1, Convert rad/s to rmp/1  "w angular speed"
  Sum1/1 -> 1/J Inertia constant/1
  Electrical Torque/1 -> Sum1/3
  Convert rad/s to rmp/1 -> "Propeller model "/1(rpm)
  "Propeller model "/2(thrust) -> Thrust/1
  staticFriction/1 -> Sum1/2

== system DJI_Quadcopter_Simulation_2018a/Quadcopter Dynamics/Motor Dynamics/Subsystem2/motorRotor4/Electrical part ==
  ESC voltage : Inport
  w angular speed : Inport  Port=2
  1/R : Gain  Gain=1/Motor.Req
  Ke (Torque constant)1 : Gain  Gain=Motor.Ke_eq
  Kt (Torque constant) Kt=Ke for an ideal square wave motor : Gain  Gain=Motor.Ke_eq
  Sum : Sum  Inputs=|+-
  Electrical Torque : Outport
  current : Outport  Port=2
  wires:
  1/R/1 -> current/1, Kt (Torque constant) Kt=Ke for an ideal square wave motor/1  "current i"
  Sum/1 -> 1/R/1
  Kt (Torque constant) Kt=Ke for an ideal square wave motor/1 -> Electrical Torque/1
  Ke (Torque constant)1/1 -> Sum/2
  ESC voltage/1 -> Sum/1
  w angular speed/1 -> Ke (Torque constant)1/1

== system DJI_Quadcopter_Simulation_2018a/Quadcopter Dynamics/Motor Dynamics/Subsystem2/motorRotor4/Mechanical part ==
  dynamicFriction : Inport
  Electrical Torque : Inport  Port=2
  1/J Inertia constant : Gain  Gain=1/Motor.J
  Convert rad/s to rmp : Gain  Gain=60/(2*pi)
  Integrator : Integrator  InitialCondition=IC.w4
  Product : Product
  "Propeller model " : MATLAB Function  TreatAsAtomicUnit=on
  Sum1 : Sum  Inputs=--+-
  staticFriction : Constant  Value=10e-7
  w angular speed : Outport
  Thrust : Outport  Port=2
  Torque : Outport  Port=3
  wires:
  "Propeller model "/1(torque) -> Sum1/1, Torque/1
  1/J Inertia constant/1 -> Integrator/1
  dynamicFriction/1 -> Product/2
  Product/1 -> Sum1/4
  Integrator/1 -> Product/1, w angular speed/1, Convert rad/s to rmp/1  "w angular speed"
  Sum1/1 -> 1/J Inertia constant/1
  Electrical Torque/1 -> Sum1/3
  Convert rad/s to rmp/1 -> "Propeller model "/1(rpm)
  "Propeller model "/2(thrust) -> Thrust/1
  staticFriction/1 -> Sum1/2

== system DJI_Quadcopter_Simulation_2018a/Quadcopter Dynamics/Motor Dynamics/Subsystem3/motorRotor4/Electrical part ==
  ESC voltage : Inport
  w angular speed : Inport  Port=2
  1/R : Gain  Gain=1/Motor.Req
  Ke (Torque constant)1 : Gain  Gain=Motor.Ke_eq
  Kt (Torque constant) Kt=Ke for an ideal square wave motor : Gain  Gain=Motor.Ke_eq
  Sum : Sum  Inputs=|+-
  Electrical Torque : Outport
  current : Outport  Port=2
  wires:
  1/R/1 -> current/1, Kt (Torque constant) Kt=Ke for an ideal square wave motor/1  "current i"
  Sum/1 -> 1/R/1
  Kt (Torque constant) Kt=Ke for an ideal square wave motor/1 -> Electrical Torque/1
  Ke (Torque constant)1/1 -> Sum/2
  ESC voltage/1 -> Sum/1
  w angular speed/1 -> Ke (Torque constant)1/1

== system DJI_Quadcopter_Simulation_2018a/Quadcopter Dynamics/Motor Dynamics/Subsystem3/motorRotor4/Mechanical part ==
  dynamicFriction : Inport
  Electrical Torque : Inport  Port=2
  1/J Inertia constant : Gain  Gain=1/Motor.J
  Convert rad/s to rmp : Gain  Gain=60/(2*pi)
  Integrator : Integrator  InitialCondition=IC.w4
  Product : Product
  "Propeller model " : MATLAB Function  TreatAsAtomicUnit=on
  Sum1 : Sum  Inputs=--+-
  staticFriction : Constant  Value=10e-7
  w angular speed : Outport
  Thrust : Outport  Port=2
  Torque : Outport  Port=3
  wires:
  "Propeller model "/1(torque) -> Sum1/1, Torque/1
  1/J Inertia constant/1 -> Integrator/1
  dynamicFriction/1 -> Product/2
  Product/1 -> Sum1/4
  Integrator/1 -> Product/1, w angular speed/1, Convert rad/s to rmp/1  "w angular speed"
  Sum1/1 -> 1/J Inertia constant/1
  Electrical Torque/1 -> Sum1/3
  Convert rad/s to rmp/1 -> "Propeller model "/1(rpm)
  "Propeller model "/2(thrust) -> Thrust/1
  staticFriction/1 -> Sum1/2
